simulink model "Aufgabe1_simu"  (Simulink 9.2)
settings: Solver=VariableStepAuto  StartTime=0.0  StopTime=10.0  RelTol=1e-3
settings Model: Creator=danial  LastModifiedBy=danial
settings DataIOCC: LimitDataPoints=off  SaveFormat=Dataset  SignalLoggingSaveFormat=Dataset
settings OptimizationCC: LifeSpan=auto
settings DebuggingCC: UnderspecifiedInitializationDetection=Simplified  MergeDetectMultiDrivingBlocksExec=error  FcnCallInpInsideContextMsg=error  StateNameClashWarn=none  SFUnexpectedBacktrackingDiag=error  SFNoUnconditionalDefaultTransitionDiag=error  SFExecutionAtInitializationDiag=warning
settings HardwareCC: ProdBitPerPointer=64  ProdBitPerSizeT=64  ProdBitPerPtrDiffT=64  ProdLargestAtomicFloat=Float  ProdIntDivRoundTo=Zero  ProdEndianess=LittleEndian  ProdWordSize=64  ProdHWDeviceType=Intel->x86-64 (Windows64)
settings ModelReferenceCC: PropagateSignalLabelsOutOfModel=on
settings SFSimCC: SimUseLocalCustomCode=on
settings RTWCC: RTWUseLocalCustomCode=on
settings CodeAppCC: StateflowObjectComments=off
settings GRTTargetCC: TargetLangStandard=C99 (ISO)  GeneratePreprocessorConditionals=Use local settings  CombineOutputUpdateFcns=on  GRTInterface=off
settings ConfigComp: CovMetricSettings=dwe  CovHtmlReporting=off  CovSaveCumulativeToWorkspaceVar=off  CovSaveSingleToWorkspaceVar=off  CovExternalEMLEnable=on

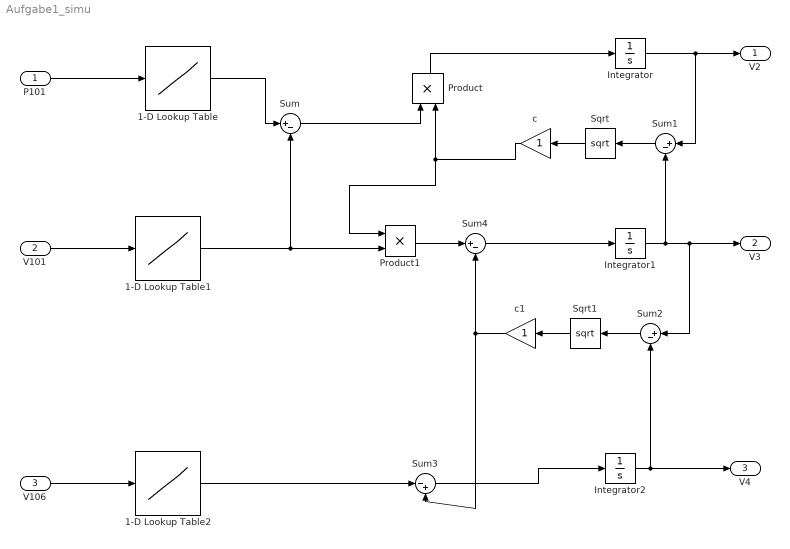
== system Aufgabe1_simu ==
  P101 : Inport
  V101 : Inport  Port=2
  V106 : Inport  Port=3
  1-D Lookup Table : Lookup_n-D  NumberOfTableDimensions=1  BreakpointsForDimension1=[-5:5]  Table=tanh([-5:5])  InternalRulePriority=Speed  RndMeth=Simplest  InputSameDT=on
  1-D Lookup Table1 : Lookup_n-D  NumberOfTableDimensions=1  BreakpointsForDimension1=[-5:5]  Table=tanh([-5:5])  InternalRulePriority=Speed  RndMeth=Simplest  InputSameDT=on
  1-D Lookup Table2 : Lookup_n-D  NumberOfTableDimensions=1  BreakpointsForDimension1=[-5:5]  Table=tanh([-5:5])  InternalRulePriority=Speed  RndMeth=Simplest  InputSameDT=on
  Integrator : Integrator
  Integrator1 : Integrator
  Integrator2 : Integrator
  Product : Product
  Product1 : Product
  Sqrt : Sqrt  SaturateOnIntegerOverflow=on
  Sqrt1 : Sqrt  SaturateOnIntegerOverflow=on
  Sum{,1..2,4} (4 alike) : Sum  Inputs=|+-
  Sum3 : Sum  Inputs=|-+
  c : Gain
  c1 : Gain
  V2 : Outport
  V3 : Outport  Port=2
  V4 : Outport  Port=3
  wires:
  P101/1 -> 1-D Lookup Table/1
  1-D Lookup Table/1 -> Sum/1
  V101/1 -> 1-D Lookup Table1/1
  V106/1 -> 1-D Lookup Table2/1
  1-D Lookup Table1/1 -> Product1/2, Sum/2
  Integrator/1 -> Sum1/1, V2/1
  Sum1/1 -> Sqrt/1
  Sqrt/1 -> c/1
  Sum/1 -> Product/1
  c/1 -> Product1/1, Product/2
  Product/1 -> Integrator/1
  Integrator1/1 -> Sum1/2, Sum2/1, V3/1
  Integrator2/1 -> V4/1, Sum2/2
  Sum2/1 -> Sqrt1/1
  Sqrt1/1 -> c1/1
  1-D Lookup Table2/1 -> Sum3/1
  c1/1 -> Sum3/2, Sum4/2
  Sum3/1 -> Integrator2/1
  Sum4/1 -> Integrator1/1
  Product1/1 -> Sum4/1
